simulink model "teste_z"  (R2020b)
settings: Solver=VariableStepAuto  StartTime=0.0  StopTime=10.0  RelTol=1e-3
settings Model: Creator=luanaraujo  LastModifiedBy=luanaraujo

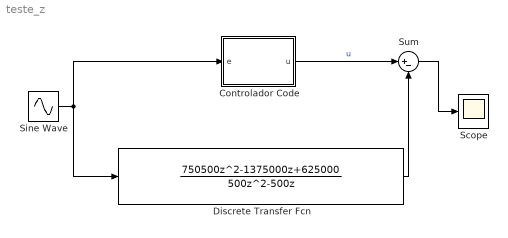
== system teste_z ==
  Controlador Code : MATLAB Function  TreatAsAtomicUnit=on
  Discrete Transfer Fcn : DiscreteTransferFcn  Numerator=[750500,-1375000,625000]  Denominator=[500,-500,0]  SampleTime=1/500
  Scope : Scope
  Sine Wave : Sin  SampleTime=1/500
  Sum : Sum  Inputs=|+-
  wires:
  Sine Wave/1 -> Discrete Transfer Fcn/1, Controlador Code/1(e)
  Controlador Code/1(u) -> Sum/1  "u"
  Discrete Transfer Fcn/1 -> Sum/2
  Sum/1 -> Scope/1

== matlab function teste_z/Controlador Code ==
  data: e input; u output
function u = fcn(e)
    persistent  sk e_1
    T = 1/500;
    kp = 250;
    ki = 500;
    kd = 2.5;
        
    if isempty(sk)
        sk = 0;
    end
    if isempty(e_1)
        e_1 = 0;
    end
    
    sk = sk + e*T; 
    saida = kp*e + (kd/T) * (e - e_1) + ki * sk;
	e_1 = e;
u = saida;
